simulink model "gm_homework1_vnl"  (R2020b)
settings: Solver=FixedStepDiscrete  StartTime=0.0  StopTime=simulation_stop_time  RelTol=1e-3
undefined symbols (not defined in the file or in its folder): sample_time
libraries: hdlsllib x8, simulink x7
settings Model: Creator=yixingli  LastModifiedBy=harsh
settings DataIOCC: LimitDataPoints=on  SaveOutput=off  SignalLogging=off  SaveTime=off
settings OptimizationCC: BlockReduction=off  ConditionallyExecuteInputs=off  DefaultParameterBehavior=Inlined  ExpressionDepthLimit=2147483647  LifeSpan=inf
settings DebuggingCC: AlgebraicLoopMsg=error  UnderspecifiedInitializationDetection=Classic  MergeDetectMultiDrivingBlocksExec=none  InheritedTsInSrcMsg=none  SingleTaskRateTransMsg=error  ParameterPrecisionLossMsg=none  AllowSymbolicDim=off  StateNameClashWarn=warning  StrictBusMsg=ErrorOnBusTreatedAsVector  SFUnexpectedBacktrackingDiag=warning  SFNoUnconditionalDefaultTransitionDiag=warning  SFExecutionAtInitializationDiag=none  ArithmeticOperatorsInVariantConditions=warning
settings HardwareCC: ProdBitPerPointer=32  ProdBitPerSizeT=32  ProdBitPerPtrDiffT=32  ProdLargestAtomicFloat=None  ProdIntDivRoundTo=Undefined  ProdEndianess=Unspecified  ProdWordSize=32  ProdHWDeviceType=ASIC/FPGA->ASIC/FPGA  ProdEqTarget=off
settings SFSimCC: SimUseLocalCustomCode=off  CustomCodeUndefinedFunction=UseInterfaceOnly
settings RTWCC: RTWUseLocalCustomCode=off
settings CodeAppCC: StateflowObjectComments=on
settings GRTTargetCC: TargetLangStandard=C89/C90 (ANSI)
settings ConfigComp: CovScope=ReferencedModels  CovMetricSettings=dw  CovSaveCumulativeToWorkspaceVar=on  CovSaveSingleToWorkspaceVar=on  CovExternalEMLEnable=off  CovSFcnEnable=off

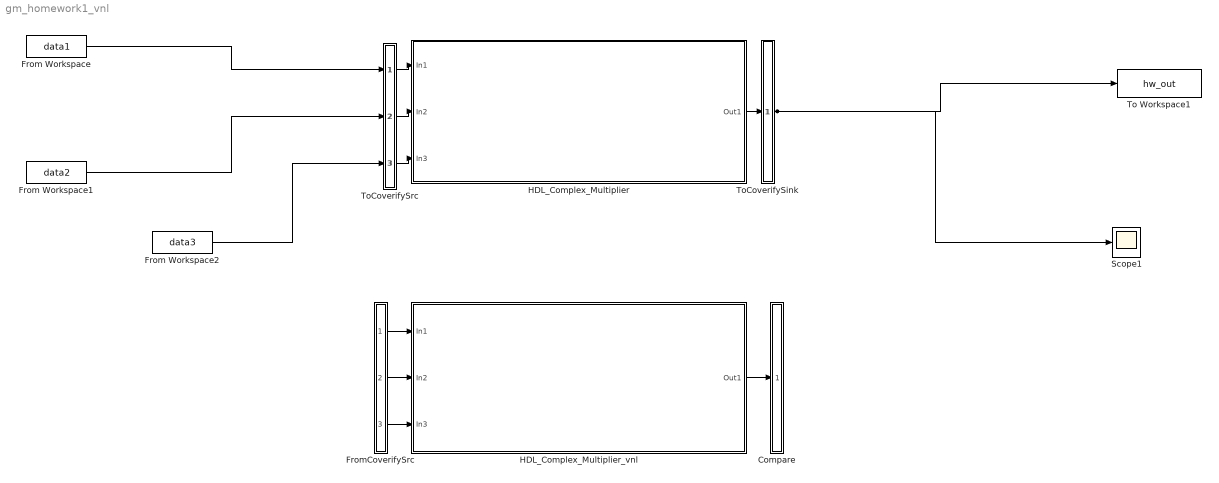
== system gm_homework1_vnl ==
  Compare : Subsystem
      mask Display: disp('')
  From Workspace : FromWorkspace  VariableName=data1  SampleTime=sample_time  Interpolate=off  OutputAfterFinalValue=Setting to zero
  From Workspace1 : FromWorkspace  VariableName=data2  SampleTime=sample_time  Interpolate=off  OutputAfterFinalValue=Setting to zero
  From Workspace2 : FromWorkspace  VariableName=data3  SampleTime=sample_time  Interpolate=off  OutputAfterFinalValue=Setting to zero
  FromCoverifySrc : Subsystem
      mask Display: disp('')
  HDL_Complex_Multiplier : Subsystem
  HDL_Complex_Multiplier_vnl : Subsystem
  Scope1 : Scope
  To Workspace1 : ToWorkspace  VariableName=hw_out  SaveFormat=Structure With Time  SampleTime=-1
  ToCoverifySink : Subsystem
      mask Display: disp('')
  ToCoverifySrc : Subsystem
      mask Display: disp('')
  wires:
  ToCoverifySrc/1(out1) -> HDL_Complex_Multiplier/1(In1)
  ToCoverifySrc/2(out2) -> HDL_Complex_Multiplier/2(In2)
  ToCoverifySrc/3(out3) -> HDL_Complex_Multiplier/3(In3)
  HDL_Complex_Multiplier/1(Out1) -> ToCoverifySink/1(in1)
  From Workspace/1 -> ToCoverifySrc/1(in1)
  From Workspace1/1 -> ToCoverifySrc/2(in2)
  From Workspace2/1 -> ToCoverifySrc/3(in3)
  ToCoverifySink/1(out1) -> Scope1/1, To Workspace1/1
  FromCoverifySrc/1(out1) -> HDL_Complex_Multiplier_vnl/1(In1)
  FromCoverifySrc/2(out2) -> HDL_Complex_Multiplier_vnl/2(In2)
  FromCoverifySrc/3(out3) -> HDL_Complex_Multiplier_vnl/3(In3)
  HDL_Complex_Multiplier_vnl/1(Out1) -> Compare/1(in1)

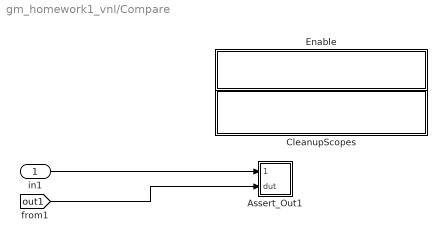
== system gm_homework1_vnl/Compare ==
  in1 : Inport
  Assert_Out1 : Subsystem
  CleanupScopes : Subsystem
      settings: OpenFcn=|
      | blkName = gcb; %self block
      | idx = regexp(blkName, '/CleanupScopes$', 'once');
      | blkParent = blkName(1:idx-1);
      | blks=find_system(blkParent, 'LookUnderMasks', 'all','blocktype', 'Scope');
      | for itr = 1:length(blks)
      | 	 hScopeCfg = get_param(blks{itr},'ScopeConfiguration');
      | 	 hScopeCfg.Visible = ~ hScopeCfg.Visible;
      | end
      | drawnow;
      mask Display: fprintf(message('hdlcoder:cosim:vnl_dblclick').getString());
  Enable : Subsystem
      settings: OpenFcn=|
      | blkName = gcb;
      | idx = regexp(blkName, '/Enable$', 'once');
      | blkParent = blkName(1:idx-1);
      | blks=find_system(blkParent, 'LookUnderMasks', 'all','blocktype', 'Assertion');
      | e = get_param(blks{1}, 'Enabled');
      | if strcmp(e, 'on'), f= 'off';, else, f = 'on';, end
      | for ii=1:length(blks), set_param(blks{ii}, 'Enabled', f);, end
      | set_param(gcb, 'MaskDisplay',['fprintf(message(''hdlcoder:cosim:vnl_dblclick_assertions'',','''',upper(e),'''',').getString())']);
      mask Display: fprintf(message('hdlcoder:cosim:vnl_dblclick_assertions','OFF').getString());
  wires:
  in1/1 -> Assert_Out1/1(cosim)
  [out1] -> Assert_Out1/2(dut)

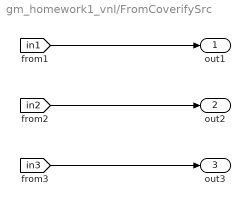
== system gm_homework1_vnl/FromCoverifySrc ==
  out1 : Outport
  out2 : Outport  Port=2
  out3 : Outport  Port=3
  wires:
  [in1] -> out1/1
  [in2] -> out2/1
  [in3] -> out3/1

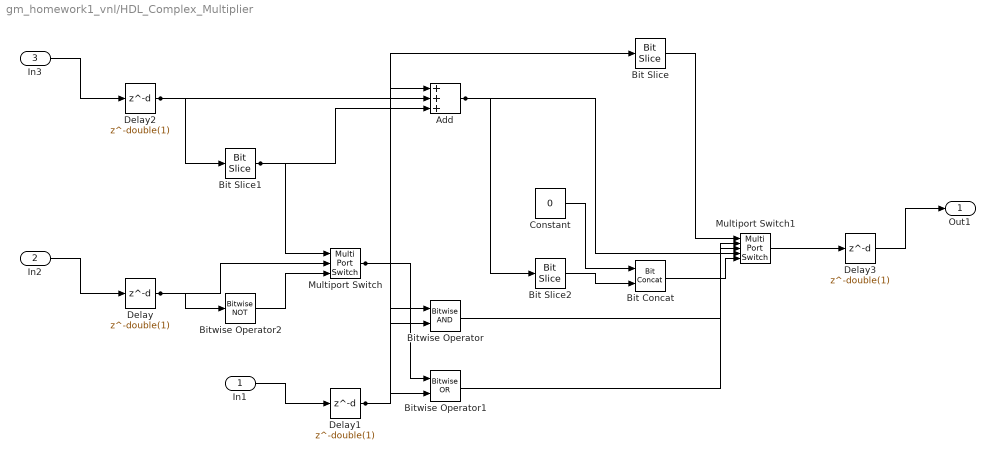
== system gm_homework1_vnl/HDL_Complex_Multiplier ==
  In1 : Inport  OutDataTypeStr=fixdt(1, 64, 0)  PortDimensions=1  SampleTime=5e-08
  In2 : Inport  Port=2  OutDataTypeStr=fixdt(1, 64, 0)  PortDimensions=1  SampleTime=5e-08
  In3 : Inport  Port=3  OutDataTypeStr=fixdt(0, 3, 0)  PortDimensions=1  SampleTime=5e-08
  Add : Sum  Inputs=+++  AccumDataTypeStr=fixdt(1, 65, 0)  OutDataTypeStr=fixdt(1, 64, 0)  SampleTime=5e-08
  Bit Concat : hdlsllib/Logic and Bit Operations/Bit Concat  numInputs=2
  Bit Slice : hdlsllib/Logic and Bit Operations/Bit Slice  lidx=double(1)  ridx=double(0)
      settings: SourceProductBaseCode=SL
  Bit Slice1 : hdlsllib/Logic and Bit Operations/Bit Slice  lidx=double(2)  ridx=double(2)
      settings: SourceProductBaseCode=SL
  Bit Slice2 : hdlsllib/Logic and Bit Operations/Bit Slice  lidx=double(62)  ridx=double(62)
      settings: SourceProductBaseCode=SL
  Bitwise Operator : simulink/Logic and Bit Operations/Bitwise Operator  logicop=AND  UseBitMask=off  NumInputPorts=2  BitMask=double(0)  BitMaskRealWorld=Real World Value
  Bitwise Operator1 : simulink/Logic and Bit Operations/Bitwise Operator  logicop=OR  UseBitMask=off  NumInputPorts=2  BitMask=double(0)  BitMaskRealWorld=Real World Value
  Bitwise Operator2 : simulink/Logic and Bit Operations/Bitwise Operator  logicop=NOT  UseBitMask=off  BitMask=double(0)  BitMaskRealWorld=Real World Value
  Constant : Constant  Value=0  OutDataTypeStr=fixdt(0, 64, 0)
  Delay{,1..3} (4 alike) : Delay  DelayLength=double(1)  InitialCondition=0  SampleTime=5e-08
  Multiport Switch : MultiPortSwitch  DataPortOrder=Zero-based contiguous  Inputs=2  DiagnosticForDefault=None  zeroidx=on  OutDataTypeStr=fixdt(1, 64, 0)  SampleTime=5e-08
  Multiport Switch1 : MultiPortSwitch  DataPortOrder=Zero-based contiguous  Inputs=4  DiagnosticForDefault=None  zeroidx=on  OutDataTypeStr=fixdt(1, 64, 0)  SampleTime=5e-08
  Out1 : Outport
  wires:
  Multiport Switch1/1 -> Delay3/1
  Multiport Switch/1 -> Add/1, Bitwise Operator/1, Bitwise Operator1/1
  Delay3/1 -> Out1/1
  Delay2/1 -> Bit Slice/1, Bit Slice1/1
  Delay1/1 -> Add/2, Bitwise Operator/2, Bitwise Operator1/2
  Delay/1 -> Bitwise Operator2/1, Multiport Switch/2
  Constant/1 -> Bit Concat/1
  Bitwise Operator2/1 -> Multiport Switch/3
  Bitwise Operator1/1 -> Multiport Switch1/3
  Bitwise Operator/1 -> Multiport Switch1/2
  Bit Slice2/1 -> Bit Concat/2
  Bit Slice1/1 -> Add/3, Multiport Switch/1
  Bit Slice/1 -> Multiport Switch1/1
  Bit Concat/1 -> Multiport Switch1/5
  Add/1 -> Bit Slice2/1, Multiport Switch1/4
  In3/1 -> Delay2/1
  In2/1 -> Delay/1
  In1/1 -> Delay1/1

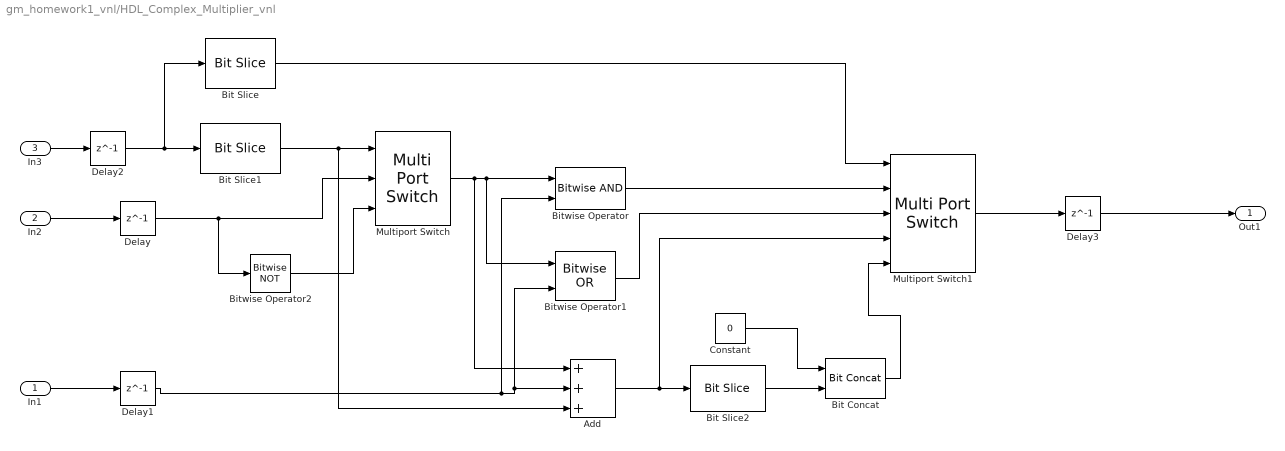
== system gm_homework1_vnl/HDL_Complex_Multiplier_vnl ==
  In1 : Inport
  In2 : Inport  Port=2
  In3 : Inport  Port=3
  Add : Sum  Inputs=+++  OutDataTypeStr=int64
  Bit Concat : hdlsllib/Logic and Bit Operations/Bit Concat  numInputs=2
  Bit Slice : hdlsllib/Logic and Bit Operations/Bit Slice  lidx=1  ridx=0
      settings: SourceProductBaseCode=SL
  Bit Slice1 : hdlsllib/Logic and Bit Operations/Bit Slice  lidx=2  ridx=2
      settings: SourceProductBaseCode=SL
  Bit Slice2 : hdlsllib/Logic and Bit Operations/Bit Slice  lidx=62  ridx=62
      settings: SourceProductBaseCode=SL
  Bitwise Operator : simulink/Logic and Bit Operations/Bitwise Operator  logicop=AND  UseBitMask=off  NumInputPorts=2  BitMask=bin2dec('11011001')  BitMaskRealWorld=Stored Integer
  Bitwise Operator1 : simulink/Logic and Bit Operations/Bitwise Operator  logicop=OR  UseBitMask=off  NumInputPorts=2  BitMask=bin2dec('11011001')  BitMaskRealWorld=Stored Integer
  Bitwise Operator2 : simulink/Logic and Bit Operations/Bitwise Operator  logicop=NOT  UseBitMask=off  BitMask=bin2dec('11011001')  BitMaskRealWorld=Stored Integer
  Constant : Constant  Value=0  OutMin=0  OutMax=63  OutDataTypeStr=uint64
  Delay{,1..3} (4 alike) : Delay  DelayLength=1  InitialCondition=0
  Multiport Switch : MultiPortSwitch  DataPortOrder=Zero-based contiguous  Inputs=2  zeroidx=on
  Multiport Switch1 : MultiPortSwitch  DataPortOrder=Zero-based contiguous  Inputs=4  zeroidx=on  OutDataTypeStr=int64
  Out1 : Outport
  wires:
  Bit Slice1/1 -> Add/3, Multiport Switch/1
  In2/1 -> Delay/1
  In1/1 -> Delay1/1
  Delay2/1 -> Bit Slice1/1, Bit Slice/1
  Bitwise Operator1/1 -> Multiport Switch1/3
  Bitwise Operator/1 -> Multiport Switch1/2
  Bit Concat/1 -> Multiport Switch1/5
  Bit Slice2/1 -> Bit Concat/2
  Constant/1 -> Bit Concat/1
  Add/1 -> Bit Slice2/1, Multiport Switch1/4
  Multiport Switch/1 -> Bitwise Operator/1, Bitwise Operator1/1, Add/1
  Delay1/1 -> Add/2, Bitwise Operator1/2, Bitwise Operator/2
  Multiport Switch1/1 -> Delay3/1
  Bit Slice/1 -> Multiport Switch1/1
  In3/1 -> Delay2/1
  Bitwise Operator2/1 -> Multiport Switch/3
  Delay/1 -> Multiport Switch/2, Bitwise Operator2/1
  Delay3/1 -> Out1/1

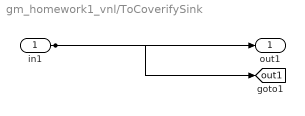
== system gm_homework1_vnl/ToCoverifySink ==
  in1 : Inport
  out1 : Outport
  tag scope: out1=global
  wires:
  in1/1 -> out1/1, [out1]

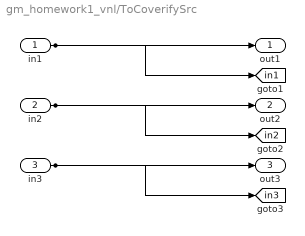
== system gm_homework1_vnl/ToCoverifySrc ==
  in1 : Inport
  in2 : Inport  Port=2
  in3 : Inport  Port=3
  out1 : Outport
  out2 : Outport  Port=2
  out3 : Outport  Port=3
  tag scope: in1=global, in2=global, in3=global
  wires:
  in1/1 -> out1/1, [in1]
  in2/1 -> out2/1, [in2]
  in3/1 -> out3/1, [in3]

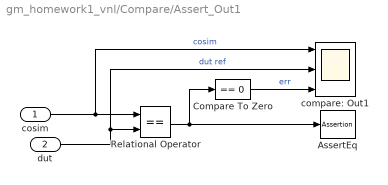
== system gm_homework1_vnl/Compare/Assert_Out1 ==
  cosim : Inport
  dut : Inport  Port=2
  AssertEq : Assertion  StopWhenAssertionFail=off
  Compare To Zero : simulink/Logic and Bit Operations/Compare To Zero  relop===  OutDataTypeStr=boolean
  Relational Operator : RelationalOperator  Operator===  OutDataTypeStr=boolean  RndMeth=Nearest
  compare: Out1 : Scope  NumInputPorts=3
  wires:
  Compare To Zero/1 -> compare: Out1/3  "err"
  Relational Operator/1 -> Compare To Zero/1, AssertEq/1
  cosim/1 -> compare: Out1/1, Relational Operator/1  "cosim"
  dut/1 -> compare: Out1/2, Relational Operator/2  "dut ref"

== system gm_homework1_vnl/Compare/CleanupScopes ==

== system gm_homework1_vnl/Compare/Enable ==
